simulink model "dsppluck"  (R2013b)
settings: Solver=FixedStepDiscrete  StartTime=0.0  StopTime=40/16  RelTol=1e-3
libraries: dspindex x2, dspmisc x1, dspsigops x1, dspbuff3 x1
CloseFcn:
  | clear y_pluck;
settings Model: ExtModeAutoUpdateStatusClock=off  Creator=The MathWorks Inc.  LastModifiedBy=tariktosun
settings DataIOCC: SignalLoggingSaveFormat=ModelDataLogs  SaveOutput=off  SaveTime=off  SignalLoggingName=sigsOut
settings OptimizationCC: ExpressionDepthLimit=2147483647  InitFltsAndDblsToZero=on
settings DebuggingCC: SaveWithParameterizedLinksMsg=none  CheckExecutionContextPreStartOutputMsg=on  CheckExecutionContextRuntimeOutputMsg=on  SignalResolutionControl=TryResolveAllWithWarning  SolverPrmCheckMsg=none  MultiTaskDSMMsg=warning  MultiTaskCondExecSysMsg=none  FcnCallInpInsideContextMsg=UseLocalSettings  StateNameClashWarn=warning
settings HardwareCC: ProdHWDeviceType=Specified
settings RTWCC: IncludeERTFirstTime=on
settings GRTTargetCC: TargetFcnLib=ansi_tfl_tmw.mat  CombineOutputUpdateFcns=off  GRTInterface=on

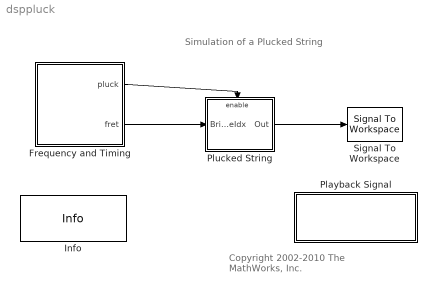
== system dsppluck ==
  note: Simulation of a Plucked String
  note: Copyright 2002-2010 The MathWorks, Inc.
  Frequency and Timing : Subsystem  mask{ptime=[0 5000 7500 10000 15000], fret=[30 14 14 23 8], Ts=1/16000}
      mask prompts: ptime "Pluck time indices:"; fret "Fret position:"; Ts "Sample time:"
      mask init:
      | % Fret position (frequency) signal
      | p=ptime(:); q=ones(size(p)).*fret(:);
      | p=p(:); q=q(:);
      | freq.time=p*Ts;
      | freq.signals.values=uint16(q);
      | freq.signals.dimensions=1;
      | 
      | % Pluck timing (enable) signal
      | p=ptime(:); p=p(2:end); q=ones(size(p));
      | p=[p p+1]'; p=[1;p(:)];
      | q=[zeros(size(q)) q]'; q=[1;q(:)];
      | ena.time=p*Ts;
      | ena.signals.values=boolean(q);
      | ena.signals.dimensions=1;
      mask Display: disp('Instrument');
  Info : dspmisc/Info  SystemSampleTime=-1
  Playback Signal : Subsystem  StopFcn=|  mask(Original Signal){}
      | if exist('y_pluck','var'),      
      |    sound(double(y_pluck),16000);
      | end
      settings: OpenFcn=|
      | if exist('y_pluck','var'),
      |    sound(double(y_pluck),16000);
      | else
      |    errordlg('Run model before playing.', ...
      |                'DSP System Toolbox Demo Error');
      | end
      mask Display: disp('Playback\nSignal')
  Plucked String : Subsystem  TreatAsAtomicUnit=on  mask(Plucked String Simulator){SLen=35, H=single(-[.25 .5 .25]), PPt=30, PickupIdx=30}
      mask prompts: SLen "String length, L (number of samples):"; H "Reflection filter (FIR):"; PPt "Pluck point, P (0 < P <= L):"; PickupIdx "Pickup index, i (0 < i <= L):"
      mask help:
      | Simulates a plucked string.  Input signal is a scalar integer value indicating the placement of the "bridge", e.g., it sets the frequency of the output.  Lower numbers lead to higher frequencies, and this must be <= L, the length of the delay line.
      |
      | String Length is a relative measure, specified in number of discrete samples, which is related to the length of the digital delay line.  It must be > 3 based on the reflection filter being used.
      |
      | Pluck Point is the position, in samples, along the string at which the displacement is centered.  This must be less than or equal to the string length.
      |
      | Pickup Index is the position,  in samples, at which the "vibration" is "sampled" to determine the output signal.
      mask init:
      | % [LtInit,RtInit] = dspblkpluck(SLen,PPt,H);
      | %
      | % pluck position is given as a sample count
      | % create triangular waveform for initialization
      | x = [ (0:floor(PPt))./PPt, ...
      |       (SLen-1-((floor(PPt)+1):(SLen-1)))./(SLen-1-PPt) ];
      | 
      | % Because initial velocity profile is flat,
      | % initial displacement profile is equal in
      | % leftgoing and rightgoing waves.
      | %
      | % Make right-going delay-line long enough to
      | % hold refl filter points centered at the end
      | % point (for calculating zero-phase reflection)
      | LtInit  = x/2;
      | RtInit = [x/2, zeros(1, length(H) - floor(length(H)/2))];
      mask Help: web(dspbhelp);
      mask Display: disp('Digital\nWaveguide\nSynthesis')
  Signal To Workspace : SignalToWorkspace  VariableName=y_pluck
      settings: CopyFcn=dspblkcopystw(gcbh);
  wires:
  Plucked String/1(Out) -> Signal To Workspace/1
  Frequency and Timing/2(fret) -> Plucked String/1(BridgeIdx)
  Frequency and Timing/1(pluck) -> Plucked String/Enable

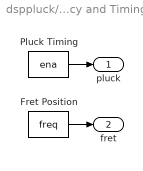
== system dsppluck/Frequency and Timing ==
  Fret Position : FromWorkspace  VariableName=freq  SampleTime=Ts  Interpolate=off  OutputAfterFinalValue=Holding final value
  Pluck Timing : FromWorkspace  VariableName=ena  SampleTime=Ts  Interpolate=off  OutputAfterFinalValue=Holding final value
  pluck : Outport
  fret : Outport  Port=2
  wires:
  Pluck Timing/1 -> pluck/1
  Fret Position/1 -> fret/1

== system dsppluck/Playback Signal ==

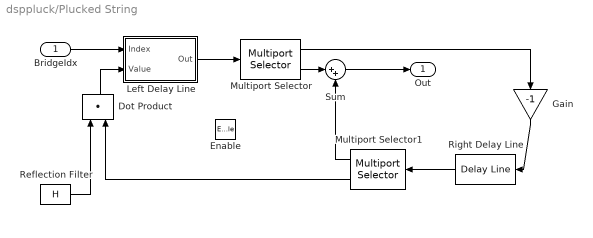
== system dsppluck/Plucked String ==
  BridgeIdx : Inport
  Enable : EnablePort  StatesWhenEnabling=reset  PropagateVarSize=During execution  ZeroCross=off
  Dot Product : DotProduct  OutDataTypeStr=Inherit: Inherit via internal rule
  Gain : Gain  Gain=-1  SaturateOnIntegerOverflow=on  OutDataTypeStr=Inherit: Same as input  ParamDataTypeStr=Inherit: Same as input
  Left Delay Line : Subsystem  mask(Variable Delay Line){siz=length(LtInit), ic=single(LtInit)}
      mask prompts: siz "Delay line size:"; ic "Initial conditions:"
      mask help:
      | Shift out delay line contents and store input data into delay line at point specified by the Index port.
      |
      | Index port expects a 1-based index.
      mask Help: web(dspbhelp);
      mask Display: disp('Variable\nDelay\nLine');
  Multiport Selector : dspindex/Multiport Selector  rowsOrCols=Rows  idxCellArray={1, PickupIdx}  idxErrMode=Clip Index
  Multiport Selector1 : dspindex/Multiport Selector  rowsOrCols=Rows  idxCellArray={PickupIdx, 1:length(H)}  idxErrMode=Clip Index
  Reflection Filter : Constant  Value=H  VectorParams1D=off
  Right Delay Line : dspbuff3/Delay Line  siz=length(RtInit)  ic=single(RtInit)  directfeed=off  enable_output=off  hold_output=off  TreatMby1Signals=One channel
  Sum : Sum  Inputs=|++  SaturateOnIntegerOverflow=on  InputSameDT=on  OutDataTypeStr=Inherit: Same as first input
  Out : Outport
  wires:
  Sum/1 -> Out/1
  BridgeIdx/1 -> Left Delay Line/1(Index)
  Dot Product/1 -> Left Delay Line/2(Value)
  Gain/1 -> Right Delay Line/1
  Multiport Selector/1 -> Gain/1
  Right Delay Line/1 -> Multiport Selector1/1
  Left Delay Line/1(Out) -> Multiport Selector/1
  Reflection Filter/1 -> Dot Product/1
  Multiport Selector/2 -> Sum/1
  Multiport Selector1/2 -> Dot Product/2
  Multiport Selector1/1 -> Sum/2

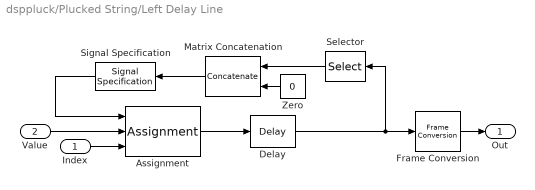
== system dsppluck/Plucked String/Left Delay Line ==
  Index : Inport
  Value : Inport  Port=2
  Assignment : Assignment  IndexOptions=Index vector (port)  Indices=1  OutputSizes=[1 1]
  Delay : dspsigops/Delay  dly_unit=Samples  delay=1  ic_detail=on  dif_ic_for_ch=on  dif_ic_for_dly=off  ic=ic  reset_popup=None
  Frame Conversion : FrameConversion
  Matrix Concatenation : Concatenate  Mode=Multidimensional array
  Selector : Selector  InputPortWidth=siz  IndexOptions=Index vector (dialog)  Indices=2:siz  OutputSizes=1
  Signal Specification : SignalSpecification  Dimensions=siz
  Zero : Constant  Value=0  VectorParams1D=off  OutDataTypeStr=Inherit: Inherit via back propagation
  Out : Outport
  wires:
  Assignment/1 -> Delay/1
  Zero/1 -> Matrix Concatenation/2
  Matrix Concatenation/1 -> Signal Specification/1
  Signal Specification/1 -> Assignment/1
  Selector/1 -> Matrix Concatenation/1
  Value/1 -> Assignment/2
  Index/1 -> Assignment/3
  Delay/1 -> Selector/1, Frame Conversion/1
  Frame Conversion/1 -> Out/1
